simulink model "reduced_order_model"  (R2015b)
settings: Solver=VariableStepAuto  StartTime=0.0  StopTime=10.0  RelTol=1e-3
values from neighbouring files (symbols this model uses):
  A = [-1 -1 0;-1 0 0;0 -1 -1]    [FULLORDERUNKNOWN.m]    (also in OBSERVER.m = [0 20.6;1 0]; functional.m = [-10 2 0 1 0; 1 -1 0 0 1;1 0 -5 3 4; -3 1 1 -8 3; -2 -4 0 2 ; lmi.m = [-10 2 0 1 0; 1 -1 0 0 1;1 0 -5 3 4; -3 1 1 -8 3; -2 -4 0 2 ; reduced_observer.m = [1 0 -2 2 0 0 -8 -6 -2;0 -1 3 18 41 -10 -19 -28 4; 1 2 3 4 4)
  B = [1;2;3]    [FULLORDERUNKNOWN.m]    (also in OBSERVER.m = [0;1]; functional.m = [1;2;3;4;5]; lmi.m = [1;2;3;4;5]; reduced_observer.m = [1;2;3;4;5;6;7;8;9])
  C = [1 0 0;0 0 1]    [FULLORDERUNKNOWN.m]    (also in OBSERVER.m = [0 1]; functional.m = [1 0 0 0 0;0 1 0 0 0]; lmi.m = [1 0 0 0 0;0 1 0 0 0]; reduced_observer.m = [1 0 0 0 0 0 0 0 0;0 1 0 0 0 0 0 0 0; 0 0 1 0 0 0 0 0 0])
  F = [1 2 0 0 1]    [functional.m]    (also in lmi.m; reduced_observer.m = A22-L*A12)
  G = G+g(i)    [functional.m]    (also in reduced_observer.m = A21-L*A11+F*L)
  H = Y*B    [FULLORDERUNKNOWN.m]    (also in reduced_observer.m = B2-L*B1)
  k = place(A,B,e)    [FULLORDERUNKNOWN.m]    (also in OBSERVER.m; functional.m = cell(Y,1); reduced_observer.m)
  L = L'    [FULLORDERUNKNOWN.m]    (also in OBSERVER.m = l'; reduced_observer.m)
  P = [pinv(C) null(C)]    [functional.m]    (also in lmi.m; reduced_observer.m)
settings Model: Creator=deepika  LastModifiedBy=deepika

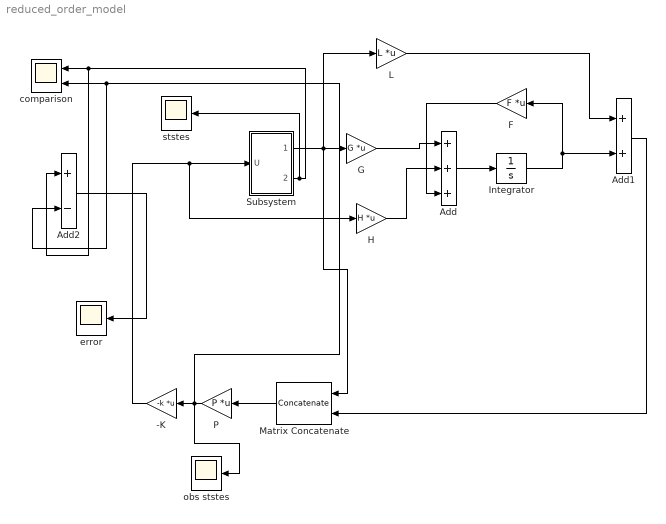
== system reduced_order_model ==
  " ststes" : Scope
  -K : Gain  Gain=-k  Multiplication=Matrix(K*u)
  Add : Sum  Inputs=+++
  Add1 : Sum
  Add2 : Sum  Inputs=+-
  F : Gain  Gain=F  Multiplication=Matrix(K*u)
  G : Gain  Gain=G  Multiplication=Matrix(K*u)
  H : Gain  Gain=H  Multiplication=Matrix(K*u)
  Integrator : Integrator  InitialCondition=[1;1;1;1;1;1]
  L : Gain  Gain=L  Multiplication=Matrix(K*u)
  Matrix Concatenate : Concatenate  ConcatenateDimension=2
  P : Gain  Gain=P  Multiplication=Matrix(K*u)
  Subsystem : Subsystem
  comparison : Scope  NumInputPorts=2
  error : Scope
  obs ststes : Scope
  wires:
  G/1 -> Add/1
  -K/1 -> H/1, Subsystem/1(U)
  H/1 -> Add/2
  Add/1 -> Integrator/1
  Integrator/1 -> Add1/2, F/1
  F/1 -> Add/3
  L/1 -> Add1/1
  Matrix Concatenate/1 -> P/1
  P/1 -> obs ststes/1, Add2/2, comparison/2, -K/1
  Add1/1 -> Matrix Concatenate/2
  Subsystem/1(OUTPUT) -> Matrix Concatenate/1, L/1, G/1
  Subsystem/2(STATES) -> " ststes"/1, Add2/1, comparison/1
  Add2/1 -> error/1

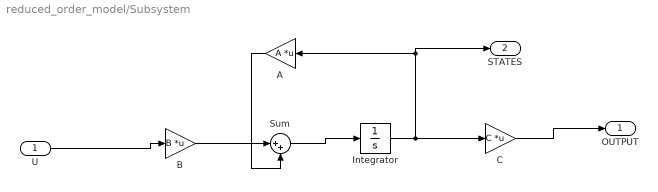
== system reduced_order_model/Subsystem ==
  U : Inport
  A : Gain  Gain=A  Multiplication=Matrix(K*u)
  B : Gain  Gain=B  Multiplication=Matrix(K*u)
  C : Gain  Gain=C  Multiplication=Matrix(K*u)
  Integrator : Integrator  InitialCondition=[1;1;1;1;1;1;1;1;1]
  Sum : Sum  Inputs=|++
  OUTPUT : Outport
  STATES : Outport  Port=2
  wires:
  B/1 -> Sum/1
  U/1 -> B/1
  Sum/1 -> Integrator/1
  Integrator/1 -> C/1, STATES/1, A/1
  A/1 -> Sum/2
  C/1 -> OUTPUT/1
